simulink model "modeloArticulo"  (R2019a)
settings: Solver=VariableStepAuto  StartTime=0.0  StopTime=30  RelTol=1e-3
libraries: simulink x1
settings Model: Creator=mluser  LastModifiedBy=mluser
settings DebuggingCC: SFMachineParentedDataDiag=error

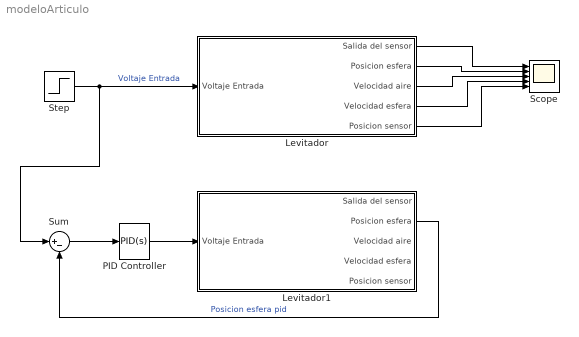
== system modeloArticulo ==
  Levitador : Subsystem
  Levitador1 : Subsystem
  PID Controller : simulink/Continuous/PID Controller  Controller=PID  Form=Parallel  TimeDomain=Continuous-time  SampleTime=-1  IntegratorMethod=Forward Euler  ControllerParametersSource=internal  P=1  I=1  D=1  UseFilter=on  N=100  TunerSelectOption=Transfer Function Based (PID Tuner App)  InitialConditionSource=internal  InitialConditionForIntegrator=0.5  InitialConditionForFilter=0  DifferentiatorICPrevScaledInput=0  ExternalReset=none  TrackingMode=off  Kt=1  LimitOutput=off  UpperSaturationLimit=inf  LowerSaturationLimit=-inf  LinearizeAsGain=on  AntiWindupMode=none  Kb=1  POutMin=[]  POutMax=[]  IOutMin=[]  IOutMax=[]  DOutMin=[]  DOutMax=[]  NOutMin=[]  NOutMax=[]  SumOutMin=[]  SumOutMax=[]  SaturationOutMin=[]  SaturationOutMax=[]  PParamMin=[]  PParamMax=[]  IParamMin=[]  IParamMax=[]  DParamMin=[]  DParamMax=[]  NParamMin=[]  NParamMax=[]  KbParamMin=[]  KbParamMax=[]  KtParamMin=[]  KtParamMax=[]  KbOutMin=[]  KbOutMax=[]  KtOutMin=[]  KtOutMax=[]  IntegratorOutMin=[]  IntegratorOutMax=[]  FilterOutMin=[]  FilterOutMax=[]  SumI1OutMin=[]  SumI1OutMax=[]  SumI2OutMin=[]  SumI2OutMax=[]  SumI3OutMin=[]  SumI3OutMax=[]  SumI4OutMin=[]  SumI4OutMax=[]  SumDOutMin=[]  SumDOutMax=[]  DifferentiatorOutMin=[]  DifferentiatorOutMax=[]  FilterDiffOutCoefMin=[]  FilterDiffOutCoefMax=[]  ReciprocalOutMin=[]  ReciprocalOutMax=[]  SumDenOutMin=[]  SumDenOutMax=[]  SumNumOutMin=[]  SumNumOutMax=[]  DivideOutMin=[]  DivideOutMax=[]  IntegratorContinuousStateAttributes=''  IntegratorStateMustResolveToSignalObject=off  IntegratorRTWStateStorageClass=Auto  FilterContinuousStateAttributes=''  FilterStateMustResolveToSignalObject=off  FilterRTWStateStorageClass=Auto  ParallelPVariant=InternalParameters  IdealPVariant=Disabled  IVariant=InternalParameters  DVariant=InternalParameters  IntegratorVariant=Continuous  SatVariant=Disabled  AWVariant=Passthrough  PCopyVariant=Disabled  TRVariant=Disabled  FdbkBlocksVariant=Forward  IdealPFdbkVariant=Disabled  SatFdbkVariant=Disabled  DerivativeFilterVariant=ContFilter  NVariant=InternalParameters  NCopyVariant=Disabled  FilterICVariant=InternalICsFilter  IntegratorICVariant=InternalICs  ExternalResetVariant=Disabled  TRSumVariant=Passthrough  SumFdbkVariant=Disabled  SumVariant=Sum_PID
  Scope : Scope  NumInputPorts=5
  Step : Step  Time=0  After=5  SampleTime=0
  Sum : Sum  Inputs=|+-
  wires:
  Levitador/1(Salida del sensor) -> Scope/1
  Levitador/2(Posicion esfera) -> Scope/2
  Levitador/3(Velocidad aire) -> Scope/3
  Levitador/4(Velocidad esfera) -> Scope/4
  Levitador/5(Posicion sensor) -> Scope/5
  Step/1 -> Sum/1, Levitador/1(Voltaje Entrada)  "Voltaje Entrada"
  Sum/1 -> PID Controller/1
  PID Controller/1 -> Levitador1/1(Voltaje Entrada)
  Levitador1/2(Posicion esfera) -> Sum/2  "Posicion esfera pid"

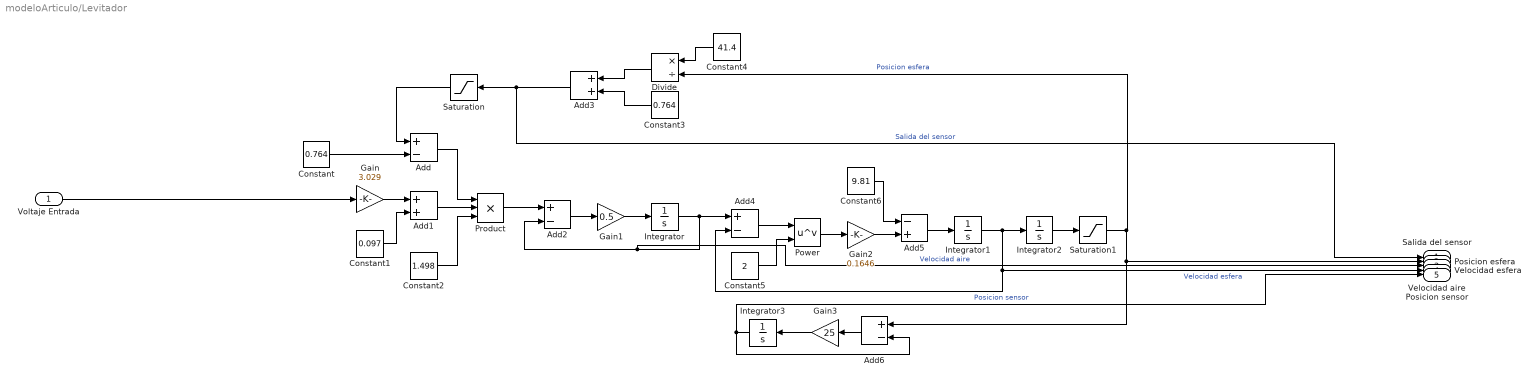
== system modeloArticulo/Levitador ==
  Voltaje Entrada : Inport
  Add{,2,4,6} (4 alike) : Sum  Inputs=+-
  Add1 : Sum
  Add3 : Sum
  Add5 : Sum  Inputs=-+
  Constant : Constant  Value=0.764
  Constant1 : Constant  Value=0.097
  Constant2 : Constant  Value=1.498
  Constant3 : Constant  Value=0.764
  Constant4 : Constant  Value=41.4
  Constant5 : Constant  Value=2
  Constant6 : Constant  Value=9.81
  Divide : Product  Inputs=*/
  Gain : Gain  Gain=3.029
  Gain1 : Gain  Gain=0.5
  Gain2 : Gain  Gain=0.1646
  Gain3 : Gain  Gain=25
  Integrator : Integrator
  Integrator1 : Integrator
  Integrator2 : Integrator  InitialCondition=0.5
  Integrator3 : Integrator
  Power : Math  Operator=pow  SaturateOnIntegerOverflow=on
  Product : Product  Inputs=3
  Saturation : Saturate  UpperLimit=2.6  LowerLimit=0.8
  Saturation1 : Saturate  UpperLimit=100  LowerLimit=0
  Salida del sensor : Outport
  Posicion esfera : Outport  Port=2
  Velocidad aire : Outport  Port=3
  Velocidad esfera : Outport  Port=4
  Posicion sensor : Outport  Port=5
  wires:
  Gain3/1 -> Integrator3/1
  Integrator2/1 -> Saturation1/1
  Add5/1 -> Integrator1/1
  Add1/1 -> Product/2
  Constant5/1 -> Power/2
  Gain/1 -> Add1/1
  Add6/1 -> Gain3/1
  Power/1 -> Gain2/1
  Add2/1 -> Gain1/1
  Integrator/1 -> Add4/1, Velocidad aire/1, Add2/2  "Velocidad aire"
  Gain2/1 -> Add5/2
  Add4/1 -> Power/1
  Product/1 -> Add2/1
  Divide/1 -> Add3/1
  Integrator3/1 -> Posicion sensor/1, Add6/2  "Posicion sensor"
  Add3/1 -> Salida del sensor/1, Saturation/1  "Salida del sensor"
  Integrator1/1 -> Integrator2/1, Velocidad esfera/1, Add4/2  "Velocidad esfera"
  Constant4/1 -> Divide/1
  Constant1/1 -> Add1/2
  Saturation1/1 -> Posicion esfera/1, Add6/1, Divide/2  "Posicion esfera"
  Saturation/1 -> Add/1
  Constant/1 -> Add/2
  Add/1 -> Product/1
  Constant3/1 -> Add3/2
  Voltaje Entrada/1 -> Gain/1
  Constant6/1 -> Add5/1
  Gain1/1 -> Integrator/1
  Constant2/1 -> Product/3

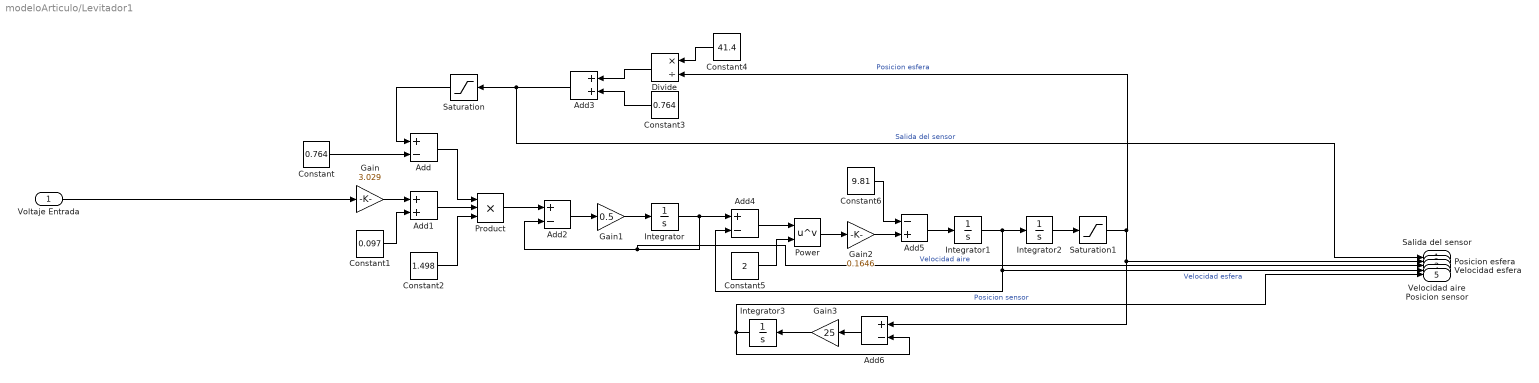
== system modeloArticulo/Levitador1 ==
  Voltaje Entrada : Inport
  Add{,2,4,6} (4 alike) : Sum  Inputs=+-
  Add1 : Sum
  Add3 : Sum
  Add5 : Sum  Inputs=-+
  Constant : Constant  Value=0.764
  Constant1 : Constant  Value=0.097
  Constant2 : Constant  Value=1.498
  Constant3 : Constant  Value=0.764
  Constant4 : Constant  Value=41.4
  Constant5 : Constant  Value=2
  Constant6 : Constant  Value=9.81
  Divide : Product  Inputs=*/
  Gain : Gain  Gain=3.029
  Gain1 : Gain  Gain=0.5
  Gain2 : Gain  Gain=0.1646
  Gain3 : Gain  Gain=25
  Integrator : Integrator
  Integrator1 : Integrator
  Integrator2 : Integrator  InitialCondition=0.5
  Integrator3 : Integrator
  Power : Math  Operator=pow  SaturateOnIntegerOverflow=on
  Product : Product  Inputs=3
  Saturation : Saturate  UpperLimit=2.6  LowerLimit=0.8
  Saturation1 : Saturate  UpperLimit=100  LowerLimit=0
  Salida del sensor : Outport
  Posicion esfera : Outport  Port=2
  Velocidad aire : Outport  Port=3
  Velocidad esfera : Outport  Port=4
  Posicion sensor : Outport  Port=5
  wires:
  Gain3/1 -> Integrator3/1
  Integrator2/1 -> Saturation1/1
  Add5/1 -> Integrator1/1
  Add1/1 -> Product/2
  Constant5/1 -> Power/2
  Gain/1 -> Add1/1
  Add6/1 -> Gain3/1
  Power/1 -> Gain2/1
  Add2/1 -> Gain1/1
  Integrator/1 -> Add4/1, Velocidad aire/1, Add2/2  "Velocidad aire"
  Gain2/1 -> Add5/2
  Add4/1 -> Power/1
  Product/1 -> Add2/1
  Divide/1 -> Add3/1
  Integrator3/1 -> Posicion sensor/1, Add6/2  "Posicion sensor"
  Add3/1 -> Salida del sensor/1, Saturation/1  "Salida del sensor"
  Integrator1/1 -> Integrator2/1, Velocidad esfera/1, Add4/2  "Velocidad esfera"
  Constant4/1 -> Divide/1
  Constant1/1 -> Add1/2
  Saturation1/1 -> Posicion esfera/1, Add6/1, Divide/2  "Posicion esfera"
  Saturation/1 -> Add/1
  Constant/1 -> Add/2
  Add/1 -> Product/1
  Constant3/1 -> Add3/2
  Voltaje Entrada/1 -> Gain/1
  Constant6/1 -> Add5/1
  Gain1/1 -> Integrator/1
  Constant2/1 -> Product/3
